simulink model "truck8_LQR00"  (Simulink 9.1)
settings: Solver=ode4  StartTime=0.0  StopTime=200  FixedStep=0.001  RelTol=1e-3  EnableMultiTasking=on
undefined symbols (not defined in the file): a1, a2, atable, atableall, cf_, cr_, den, dpsi, integrator_saturation_level1, integrator_saturation_level2, iz_, Kc, Kforward, Ki, ki1, ki2, KK1, KK2, KK3, KK4, KK_m2table, KK_vtable, Klon, kp1, kp2, Ksteer, lf_, londelay, lr_, m2, mass_, num, PP0, PP1, PP2, PP3, PP_m2table, PP_vtable, query_time, speed_controller_input_limit, st1, station_error_limit, steer0, steerdelay, t1, t2, Tlon, Tr, Tsteer, utable, utableall, v, vtable, wheelbase_
libraries: simulink x8, Solver_SF x1
settings Model: Creator=CIDI_xuhao  LastModifiedBy=DELL  SimulationMode=rapid-accelerator
settings DataIOCC: SaveFormat=Dataset
settings DebuggingCC: UnderspecifiedInitializationDetection=Simplified  MergeDetectMultiDrivingBlocksExec=error
settings HardwareCC: ProdBitPerPointer=64  ProdBitPerSizeT=64  ProdBitPerPtrDiffT=64  ProdLargestAtomicFloat=Float  ProdIntDivRoundTo=Zero  ProdEndianess=LittleEndian  ProdWordSize=64  ProdHWDeviceType=Intel->x86-64 (Windows64)
settings ModelReferenceCC: PropagateSignalLabelsOutOfModel=on
settings GRTTargetCC: GeneratePreprocessorConditionals=Disable all  CombineOutputUpdateFcns=on  GRTInterface=off

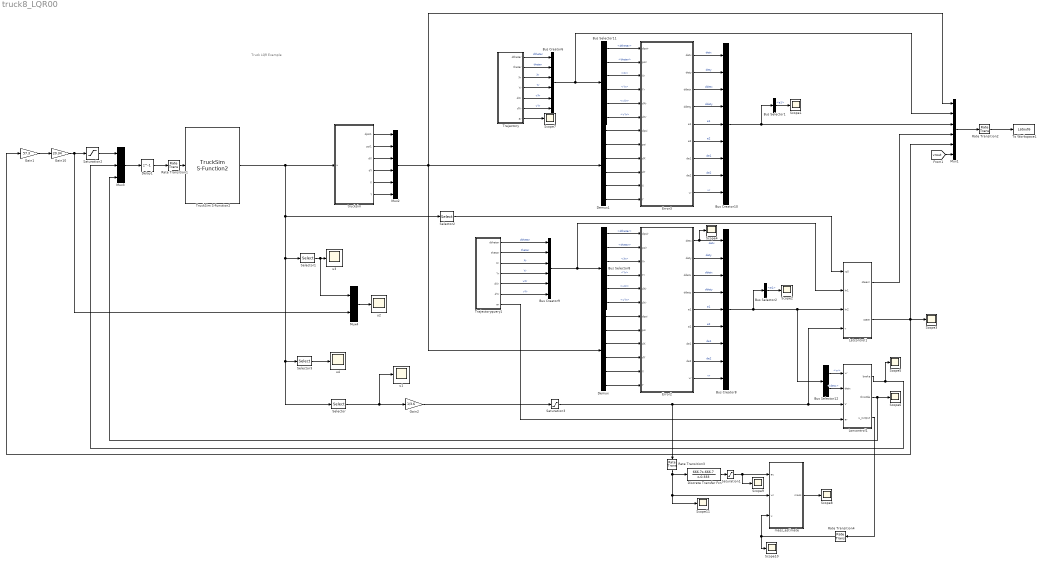
== system truck8_LQR00 ==
  note: Truck LQR Example
  Bus Creator10 : BusCreator  Inputs=9
  Bus Creator6 : BusCreator  Inputs=6
  Bus Creator8 : BusCreator  Inputs=9
  Bus Creator9 : BusCreator  Inputs=6
  Bus Selector1 : BusSelector  OutputSignals=e1
  Bus Selector11 : BusSelector  OutputSignals=dthetar,thetar,Xr,Yr,vXr,vYr
  Bus Selector12 : BusSelector  OutputSignals=vr,detx
  Bus Selector2 : BusSelector  OutputSignals=e1
  Bus Selector8 : BusSelector  OutputSignals=dthetar,thetar,Xr,Yr,vXr,vYr
  Delay1 : Delay  DelayLength=1  InitialCondition=0
  Demux : Demux  Outputs=6
  Demux1 : Demux  Outputs=6
  Discrete Transfer Fcn : DiscreteTransferFcn  Numerator=[666.7 -666.7]  Denominator=[1 -0.333]
  Error2 : MATLAB Function  TreatAsAtomicUnit=on
  Error3 : MATLAB Function  TreatAsAtomicUnit=on
  Gain1 : Gain  Gain=57.3
  Gain10 : Gain  Gain=20.34
  Gain2 : Gain  Gain=1/3.6
  Latcontrol1 : Subsystem
  Loncontrol1 : Subsystem
  Mux1 : Mux  Inputs=6
  Mux2 : Mux  Inputs=6
  Mux3 : Mux  Inputs=3
  Mux4 : Mux  Inputs=2
  Rate Transition1 : RateTransition  OutPortSampleTime=0.001
  Rate Transition2 : RateTransition  OutPortSampleTime=0.01
  Rate Transition3 : RateTransition  OutPortSampleTime=0.01
  Rate Transition4 : RateTransition  OutPortSampleTime=0.01
  Saturation1 : Saturate  UpperLimit=2  LowerLimit=-2
  Saturation2 : Saturate  UpperLimit=800  LowerLimit=-800
  Saturation3 : Saturate  UpperLimit=inf  LowerLimit=0.1
  Scope{1..11} (11 alike) : Scope
  Selector : Selector  InputPortWidth=13  IndexOptions=Index vector (dialog)  Indices=[4]  OutputSizes=1
  Selector1 : Selector  InputPortWidth=13  IndexOptions=Index vector (dialog)  Indices=[11 12]  OutputSizes=1
  Selector2 : Selector  InputPortWidth=13  IndexOptions=Index vector (dialog)  Indices=[11]  OutputSizes=1
  Selector3 : Selector  InputPortWidth=13  IndexOptions=Index vector (dialog)  Indices=[13]  OutputSizes=1
  To Workspace1 : ToWorkspace  VariableName=Latout6  SaveFormat=Timeseries  SampleTime=-1
  Trajectory : Subsystem
  Trajectoryquery1 : Subsystem
  TruckSim S-Function2 : Solver_SF/TruckSim S-Function2  Priority=1  VehicleCode=s_ss__sss  SIMFILE=simfile.sim
      settings: AttributesFormatString=Vehicle Code: %<VehicleCode>
  mass_estimate : Subsystem
  trucksim : MATLAB Function  TreatAsAtomicUnit=on
  u{1..4} (4 alike) : Scope
  wires:
  Selector/1 -> u1/1, Gain2/1
  Error2/7(de1) -> Bus Creator8/7  "de1"
  Trajectory/4(Yr) -> Bus Creator6/4  "Yr"
  Error2/3(ddetx) -> Bus Creator8/3  "ddetx"
  Bus Selector11/5 -> Error3/5(dXr)  "<vXr>"
  Demux/4 -> Error2/10(dY)
  Trajectoryquery1/1(dthetar) -> Bus Creator9/1  "dthetar"
  Error3/8(de2) -> Bus Creator10/8  "de2"
  Demux/1 -> Error2/7(dpsi)
  Error3/7(de1) -> Bus Creator10/7  "de1"
  Trajectoryquery1/5(dXr) -> Bus Creator9/5  "vXr"
  Bus Selector11/6 -> Error3/6(dYr)  "<vYr>"
  Bus Creator10/1 -> Bus Selector1/1, Mux1/3
  Error3/4(ddety) -> Bus Creator10/4  "ddety"
  Bus Selector12/1 -> Loncontrol1/1(vr)  "<vr>"
  Bus Selector11/3 -> Error3/3(Xr)  "<Xr>"
  Bus Selector11/2 -> Error3/2(psir)  "<thetar>"
  Demux1/6 -> Error3/12(Y)
  Bus Selector11/4 -> Error3/4(Yr)  "<Yr>"
  Error3/3(ddetx) -> Bus Creator10/3  "ddetx"
  Bus Selector12/2 -> Loncontrol1/2(detx)  "<detx>"
  Demux1/1 -> Error3/7(dpsi)
  [vrout] -> Mux1/6
  Bus Selector11/1 -> Error3/1(dpsir)  "<dthetar>"
  Demux1/5 -> Error3/11(X)
  Trajectoryquery1/6(dYr) -> Bus Creator9/6  "vYr"
  Error3/2(dety) -> Bus Creator10/2  "dety"
  Bus Selector8/2 -> Error2/2(psir)  "<thetar>"
  Error3/1(detx) -> Bus Creator10/1  "detx"
  Error2/5(e1) -> Bus Creator8/5  "e1"
  Demux/6 -> Error2/12(Y)
  Error3/6(e2) -> Bus Creator10/6  "e2"
  Error2/6(e2) -> Bus Creator8/6  "e2"
  Error3/9(vr) -> Bus Creator10/9  "vr"
  Demux/2 -> Error2/8(psi)
  Error2/2(dety) -> Bus Creator8/2  "dety"
  Error2/9(vr) -> Bus Creator8/9  "vr"
  Latcontrol1/1(steerc) -> Mux1/4
  Bus Selector8/3 -> Error2/3(Xr)  "<Xr>"
  Trajectoryquery1/2(thetar) -> Bus Creator9/2  "thetar"
  Bus Selector8/4 -> Error2/4(Yr)  "<Yr>"
  Bus Selector8/5 -> Error2/5(dXr)  "<vXr>"
  Error2/8(de2) -> Bus Creator8/8  "de2"
  Trajectory/5(dXr) -> Bus Creator6/5  "vXr"
  Trajectory/3(Xr) -> Bus Creator6/3  "Xr"
  Trajectory/6(dYr) -> Bus Creator6/6  "vYr"
  Trajectory/2(thetar) -> Bus Creator6/2  "thetar"
  Demux/3 -> Error2/9(dX)
  Bus Selector8/6 -> Error2/6(dYr)  "<vYr>"
  Error3/5(e1) -> Bus Creator10/5  "e1"
  Error2/1(detx) -> Bus Creator8/1, Scope4/1  "detx"
  Error2/4(ddety) -> Bus Creator8/4  "ddety"
  Mux1/1 -> Rate Transition2/1
  Bus Selector8/1 -> Error2/1(dpsir)  "<dthetar>"
  Trajectoryquery1/3(Xr) -> Bus Creator9/3  "Xr"
  Demux/5 -> Error2/11(X)
  Trajectoryquery1/4(Yr) -> Bus Creator9/4  "Yr"
  Trajectory/1(dthetar) -> Bus Creator6/1  "dthetar"
  Rate Transition2/1 -> To Workspace1/1
  Rate Transition1/1 -> TruckSim S-Function2/1
  trucksim/1(dpsi1) -> Mux2/1
  trucksim/2(psi1) -> Mux2/2
  trucksim/3(dX) -> Mux2/3
  trucksim/4(dY) -> Mux2/4
  trucksim/5(X) -> Mux2/5
  trucksim/6(Y) -> Mux2/6
  Demux1/2 -> Error3/8(psi)
  Demux1/3 -> Error3/9(dX)
  Demux1/4 -> Error3/10(dY)
  Bus Creator6/1 -> Bus Selector11/1, Mux1/2
  Mux2/1 -> Demux/1, Demux1/1, Mux1/1
  Selector1/1 -> Mux4/1, u3/1
  Bus Selector1/1 -> Scope1/1  "<e1>"
  Mux3/1 -> Delay1/1
  Loncontrol1/2(throttle) -> Scope6/1, Mux3/3
  Gain2/1 -> Saturation3/1
  Delay1/1 -> Rate Transition1/1
  Bus Selector2/1 -> Scope2/1  "<e1>"
  Loncontrol1/1(brake) -> Scope5/1, Mux3/2
  Trajectoryquery1/7(ar) -> Loncontrol1/4(ar)
  Trajectory/7(ar) -> Scope7/1
  TruckSim S-Function2/1 -> trucksim/1(u), Selector1/1, Selector3/1, Selector/1, Selector2/1
  Bus Creator9/1 -> Latcontrol1/2(In1), Bus Selector8/1
  Saturation3/1 -> Latcontrol1/4(v), Loncontrol1/3(V), Rate Transition3/1
  Bus Creator8/1 -> Latcontrol1/3(In2), Bus Selector12/1, Bus Selector2/1
  Latcontrol1/2(steer) -> Gain1/1, Scope3/1, Mux1/5
  Gain1/1 -> Gain10/1
  Gain10/1 -> Mux4/2, Saturation2/1
  Saturation2/1 -> Mux3/1
  Mux4/1 -> u2/1
  Selector2/1 -> Latcontrol1/1(roll)
  Selector3/1 -> u4/1
  mass_estimate/1(mass) -> Scope8/1
  Rate Transition3/1 -> Discrete Transfer Fcn/1, Scope11/1, mass_estimate/2(vc)
  Discrete Transfer Fcn/1 -> Saturation1/1
  Loncontrol1/3(u_output) -> Rate Transition4/1
  Rate Transition4/1 -> mass_estimate/3(u), Scope10/1
  Saturation1/1 -> Scope9/1, mass_estimate/1(ac)

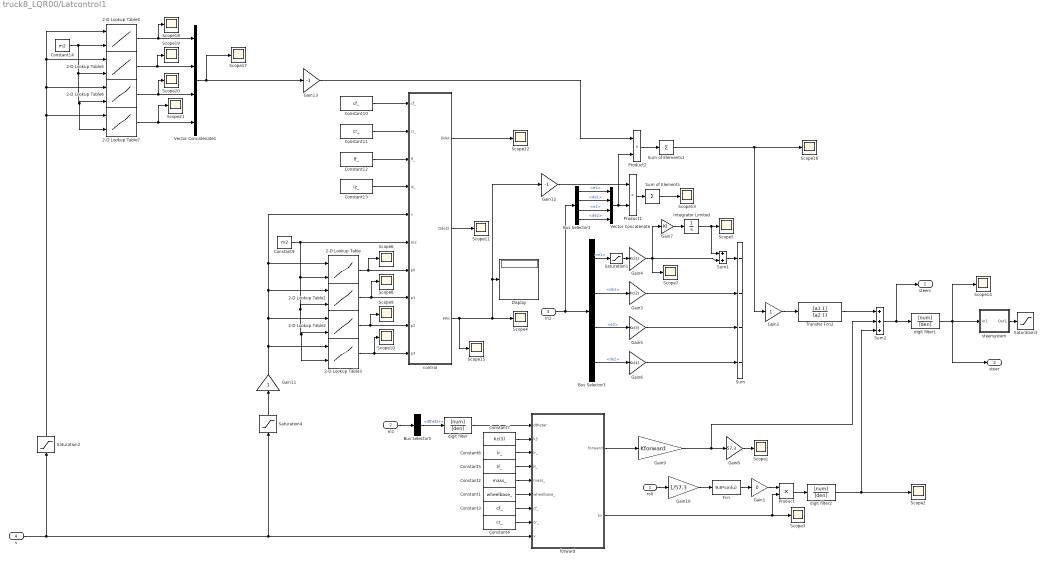
== system truck8_LQR00/Latcontrol1 ==
  roll : Inport
  In1 : Inport  Port=2
  In2 : Inport  Port=3
  v : Inport  Port=4
  2-D Lookup Table : Lookup_n-D  BreakpointsForDimension1=PP_vtable  BreakpointsForDimension2=PP_m2table  Table=PP0  ExtrapMethod=Clip  InternalRulePriority=Speed  RndMeth=Simplest  InputSameDT=on
  2-D Lookup Table1 : Lookup_n-D  BreakpointsForDimension1=PP_vtable  BreakpointsForDimension2=PP_m2table  Table=PP1  ExtrapMethod=Clip  InternalRulePriority=Speed  RndMeth=Simplest  InputSameDT=on
  2-D Lookup Table2 : Lookup_n-D  BreakpointsForDimension1=PP_vtable  BreakpointsForDimension2=PP_m2table  Table=PP2  ExtrapMethod=Clip  InternalRulePriority=Speed  RndMeth=Simplest  InputSameDT=on
  2-D Lookup Table3 : Lookup_n-D  BreakpointsForDimension1=PP_vtable  BreakpointsForDimension2=PP_m2table  Table=PP3  ExtrapMethod=Clip  InternalRulePriority=Speed  RndMeth=Simplest  InputSameDT=on
  2-D Lookup Table4 : Lookup_n-D  BreakpointsForDimension1=KK_vtable  BreakpointsForDimension2=KK_m2table  Table=KK1  ExtrapMethod=Clip  InternalRulePriority=Speed  RndMeth=Simplest  InputSameDT=on
  2-D Lookup Table5 : Lookup_n-D  BreakpointsForDimension1=KK_vtable  BreakpointsForDimension2=KK_m2table  Table=KK2  ExtrapMethod=Clip  InternalRulePriority=Speed  RndMeth=Simplest  InputSameDT=on
  2-D Lookup Table6 : Lookup_n-D  BreakpointsForDimension1=KK_vtable  BreakpointsForDimension2=KK_m2table  Table=KK3*1  ExtrapMethod=Clip  InternalRulePriority=Speed  RndMeth=Simplest  InputSameDT=on
  2-D Lookup Table7 : Lookup_n-D  BreakpointsForDimension1=KK_vtable  BreakpointsForDimension2=KK_m2table  Table=KK4  ExtrapMethod=Clip  InternalRulePriority=Speed  RndMeth=Simplest  InputSameDT=on
  Bus Selector1 : BusSelector  OutputSignals=e1,de1,e2,de2
  Bus Selector3 : BusSelector  OutputSignals=e1,de1,e2,de2
  Bus Selector5 : BusSelector  OutputSignals=dthetar
  Constant1 : Constant  Value=wheelbase_
  Constant10 : Constant  Value=cf_
  Constant11 : Constant  Value=cr_
  Constant12 : Constant  Value=lf_
  Constant13 : Constant  Value=iz_
  Constant14 : Constant  Value=m2
  Constant2 : Constant  Value=mass_
  Constant3 : Constant  Value=cf_
  Constant4 : Constant  Value=cr_
  Constant5 : Constant  Value=lf_
  Constant6 : Constant  Value=lr_
  Constant7 : Constant  Value=Kc(3)
  Constant9 : Constant  Value=m2
  Display : Display
  Fcn : Fcn  Expr=9.8*sin(u)
  Gain1 : Gain  Gain=0
  Gain10 : Gain  Gain=1/57.3
  Gain11 : Gain
  Gain12 : Gain  Gain=-1
  Gain13 : Gain  Gain=-1
  Gain2 : Gain
  Gain3 : Gain  Gain=Kc(2)
  Gain4 : Gain  Gain=Kc(1)
  Gain5 : Gain  Gain=Kc(3)
  Gain6 : Gain  Gain=Kc(4)
  Gain7 : Gain  Gain=Ki
  Gain8 : Gain  Gain=57.3
  Gain9 : Gain  Gain=Kforward
  Integrator Limited : Integrator  LimitOutput=on  UpperSaturationLimit=1  LowerSaturationLimit=-1
  Product : Product
  Product1 : Product
  Product2 : Product
  Saturation1 : Saturate  UpperLimit=10  LowerLimit=-10
  Saturation2 : Saturate  UpperLimit=25  LowerLimit=5/3.6
  Saturation3 : Saturate  UpperLimit=30/57.3  LowerLimit=-30/57.3
  Saturation4 : Saturate  UpperLimit=25  LowerLimit=10/3.6
  Scope{1..21} (21 alike) : Scope
  Sum : Sum  Inputs=----
  Sum of Elements : Sum  Inputs=+
  Sum of Elements1 : Sum  Inputs=+
  Sum1 : Sum
  Sum2 : Sum  Inputs=+++
  Transfer Fcn2 : TransferFcn  Numerator=[a1 1]  Denominator=[a2 1]
  Vector Concatenate : Concatenate  NumInputs=4
  Vector Concatenate1 : Concatenate  NumInputs=4
  control : MATLAB Function  TreatAsAtomicUnit=on
  digit filter : TransferFcn  Numerator=[num]  Denominator=[den]
  digit filter1 : TransferFcn  Numerator=[num]  Denominator=[den]
  digit filter2 : TransferFcn  Numerator=[num]  Denominator=[den]
  forward : MATLAB Function  TreatAsAtomicUnit=on
  steersystem : Subsystem
  steerc : Outport
  steer : Outport  Port=2
  wires:
  v/1 -> Saturation2/1, forward/9(v), Saturation4/1
  In2/1 -> Bus Selector1/1, Bus Selector3/1
  Bus Selector5/1 -> digit filter/1  "<dthetar>"
  In1/1 -> Bus Selector5/1
  Constant7/1 -> forward/2(k3)
  Gain8/1 -> Scope1/1
  forward/1(forward) -> Gain9/1
  Constant3/1 -> forward/7(cf_)
  Constant6/1 -> forward/3(lr_)
  Constant5/1 -> forward/4(lf_)
  Gain9/1 -> Sum2/2, Gain8/1
  Constant4/1 -> forward/8(cr_)
  steersystem/1(Out1) -> Saturation3/1
  Constant2/1 -> forward/5(mass_)
  Bus Selector3/2 -> Gain3/1  "<de1>"
  Bus Selector3/3 -> Gain5/1  "<e2>"
  Sum1/1 -> Sum/1
  Bus Selector3/1 -> Saturation1/1  "<e1>"
  Saturation1/1 -> Gain4/1
  Gain6/1 -> Sum/4
  Gain5/1 -> Sum/3
  Integrator Limited/1 -> Sum1/1, Scope5/1
  Gain4/1 -> Sum1/2, Scope7/1, Gain7/1
  Bus Selector3/4 -> Gain6/1  "<de2>"
  Constant1/1 -> forward/6(wheelbase_)
  Gain3/1 -> Sum/2
  Gain7/1 -> Integrator Limited/1
  digit filter/1 -> forward/1(dthetar)
  Gain2/1 -> Transfer Fcn2/1
  Sum2/1 -> steerc/1, digit filter1/1
  digit filter1/1 -> Scope14/1, steer/1, steersystem/1(In1)
  roll/1 -> Gain10/1
  Fcn/1 -> Gain1/1
  Gain10/1 -> Fcn/1
  digit filter2/1 -> Scope2/1, Sum2/3
  Gain1/1 -> Product/1
  Product/1 -> digit filter2/1
  forward/2(kv) -> Scope3/1, Product/2
  Transfer Fcn2/1 -> Sum2/1
  Constant12/1 -> control/3(lf_)
  Constant9/1 -> 2-D Lookup Table3/2, 2-D Lookup Table2/2, 2-D Lookup Table1/2, 2-D Lookup Table/2, control/6(m2)
  Constant10/1 -> control/1(cf_)
  Constant11/1 -> control/2(cr_)
  Constant13/1 -> control/4(iz_)
  2-D Lookup Table/1 -> Scope6/1, control/7(p0)
  2-D Lookup Table1/1 -> Scope8/1, control/8(p1)
  2-D Lookup Table3/1 -> Scope10/1, control/10(p3)
  Gain11/1 -> control/5(v), 2-D Lookup Table/1, 2-D Lookup Table1/1, 2-D Lookup Table2/1, 2-D Lookup Table3/1
  2-D Lookup Table2/1 -> Scope9/1, control/9(p2)
  Saturation4/1 -> Gain11/1
  control/2(Ddet2) -> Scope11/1
  control/1(Ddet) -> Scope12/1
  Bus Selector1/1 -> Vector Concatenate/1  "<e1>"
  Bus Selector1/2 -> Vector Concatenate/2  "<de1>"
  Bus Selector1/3 -> Vector Concatenate/3  "<e2>"
  Bus Selector1/4 -> Vector Concatenate/4  "<de2>"
  Vector Concatenate/1 -> Product2/2, Product1/2
  Product1/1 -> Sum of Elements/1
  Sum of Elements/1 -> Scope13/1
  Gain12/1 -> Product1/1
  control/3(PPK) -> Gain12/1, Display/1, Scope4/1, Scope15/1
  Saturation2/1 -> 2-D Lookup Table7/1, 2-D Lookup Table6/1, 2-D Lookup Table5/1, 2-D Lookup Table4/1
  2-D Lookup Table4/1 -> Scope18/1, Vector Concatenate1/1
  Constant14/1 -> 2-D Lookup Table4/2, 2-D Lookup Table5/2, 2-D Lookup Table7/2, 2-D Lookup Table6/2
  2-D Lookup Table5/1 -> Scope19/1, Vector Concatenate1/2
  2-D Lookup Table6/1 -> Scope20/1, Vector Concatenate1/3
  2-D Lookup Table7/1 -> Scope21/1, Vector Concatenate1/4
  Product2/1 -> Sum of Elements1/1
  Vector Concatenate1/1 -> Scope17/1, Gain13/1
  Sum of Elements1/1 -> Scope16/1, Gain2/1
  Gain13/1 -> Product2/1

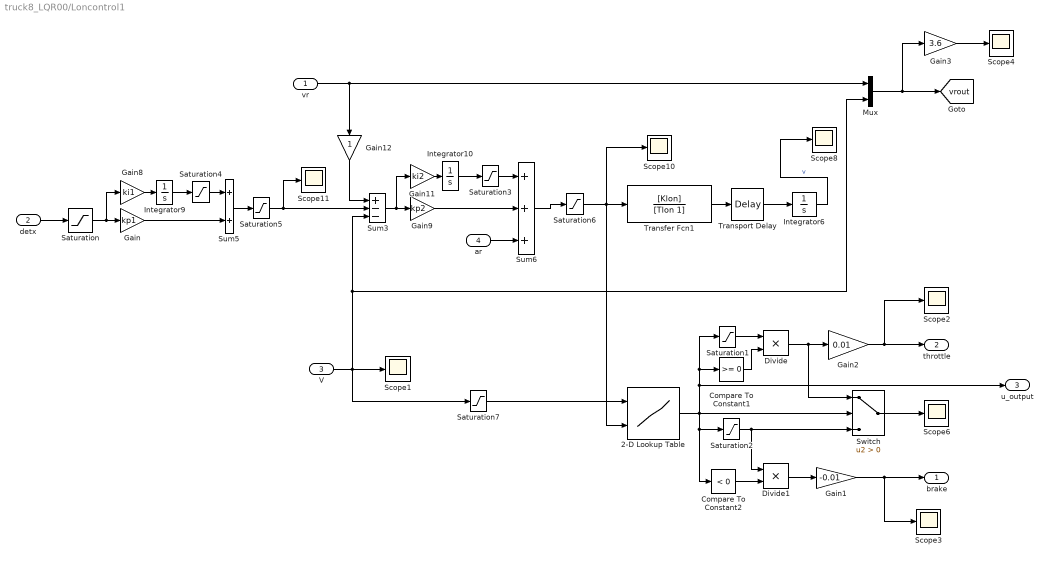
== system truck8_LQR00/Loncontrol1 ==
  vr : Inport
  detx : Inport  Port=2
  V : Inport  Port=3
  ar : Inport  Port=4
  2-D Lookup Table : Lookup_n-D  BreakpointsForDimension1=vtable  BreakpointsForDimension2=atable  Table=utableall  ExtrapMethod=Clip  InternalRulePriority=Speed  RndMeth=Simplest  InputSameDT=on
  Compare To Constant1 : simulink/Logic and Bit Operations/Compare To Constant  relop=>=  const=0  OutDataTypeStr=boolean
  Compare To Constant2 : simulink/Logic and Bit Operations/Compare To Constant  relop=<  const=0  OutDataTypeStr=boolean
  Divide : Product  Inputs=**
  Divide1 : Product  Inputs=**
  Gain : Gain  Gain=kp1
  Gain1 : Gain  Gain=-0.01
  Gain11 : Gain  Gain=ki2
  Gain12 : Gain
  Gain2 : Gain  Gain=0.01
  Gain3 : Gain  Gain=3.6
  Gain8 : Gain  Gain=ki1
  Gain9 : Gain  Gain=kp2
  Integrator10 : Integrator
  Integrator6 : Integrator
  Integrator9 : Integrator
  Mux : Mux  Inputs=2
  Saturation : Saturate  UpperLimit=station_error_limit  LowerLimit=-station_error_limit
  Saturation1 : Saturate  UpperLimit=90  LowerLimit=40*0.2
  Saturation2 : Saturate  UpperLimit=-30*0.2  LowerLimit=-60
  Saturation3 : Saturate  UpperLimit=integrator_saturation_level2  LowerLimit=-integrator_saturation_level2
  Saturation4 : Saturate  UpperLimit=integrator_saturation_level1  LowerLimit=-integrator_saturation_level1
  Saturation5 : Saturate  UpperLimit=speed_controller_input_limit  LowerLimit=-speed_controller_input_limit
  Saturation6 : Saturate  UpperLimit=5  LowerLimit=-5
  Saturation7 : Saturate  UpperLimit=100  LowerLimit=0.1
  Scope{1..4,6,8,10..11} (8 alike) : Scope
  Sum3 : Sum  Inputs=+--
  Sum5 : Sum
  Sum6 : Sum  Inputs=+++
  Switch : Switch  Criteria=u2 > Threshold
  Transfer Fcn1 : TransferFcn  Numerator=[Klon]  Denominator=[Tlon 1]
  Transport Delay : TransportDelay  DelayTime=londelay
  brake : Outport
  throttle : Outport  Port=2
  u_output : Outport  Port=3
  tag scope: vrout=global
  wires:
  Mux/1 -> Gain3/1, [vrout]
  detx/1 -> Saturation/1
  Integrator9/1 -> Saturation4/1
  Saturation3/1 -> Sum6/1
  Gain9/1 -> Sum6/2
  vr/1 -> Gain12/1, Mux/1
  Sum3/1 -> Gain11/1, Gain9/1
  Saturation/1 -> Gain/1, Gain8/1
  Gain8/1 -> Integrator9/1
  Saturation6/1 -> 2-D Lookup Table/2, Transfer Fcn1/1, Scope10/1
  Gain11/1 -> Integrator10/1
  Saturation5/1 -> Scope11/1, Sum3/2
  Gain/1 -> Sum5/2
  Integrator10/1 -> Saturation3/1
  Gain12/1 -> Sum3/1
  Saturation4/1 -> Sum5/1
  Transfer Fcn1/1 -> Transport Delay/1
  Sum5/1 -> Saturation5/1
  Transport Delay/1 -> Integrator6/1
  V/1 -> Sum3/3, Mux/2, Saturation7/1, Scope1/1
  Saturation2/1 -> Divide1/1, Switch/3
  Sum6/1 -> Saturation6/1
  Switch/1 -> Scope6/1
  Integrator6/1 -> Scope8/1  "v"
  Saturation7/1 -> 2-D Lookup Table/1
  Gain2/1 -> Scope2/1, throttle/1
  Gain1/1 -> Scope3/1, brake/1
  2-D Lookup Table/1 -> u_output/1, Compare To Constant1/1, Saturation1/1, Switch/2, Compare To Constant2/1, Saturation2/1
  Saturation1/1 -> Divide/1
  Compare To Constant1/1 -> Divide/2
  Divide/1 -> Gain2/1, Switch/1
  Compare To Constant2/1 -> Divide1/2
  Divide1/1 -> Gain1/1
  ar/1 -> Sum6/3
  Gain3/1 -> Scope4/1

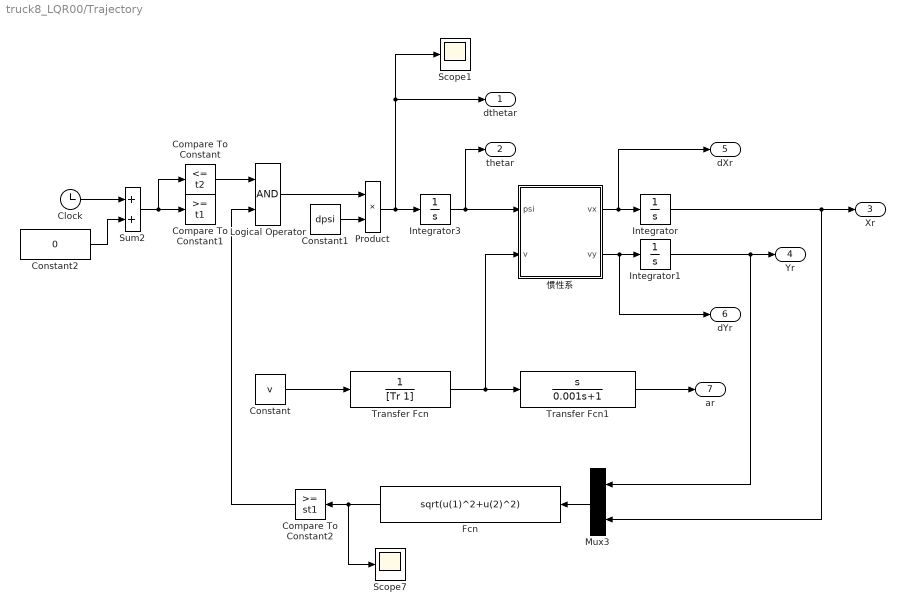
== system truck8_LQR00/Trajectory ==
  Clock : Clock
  Compare To Constant : simulink/Logic and Bit Operations/Compare To Constant  relop=<=  const=t2  OutDataTypeStr=boolean
  Compare To Constant1 : simulink/Logic and Bit Operations/Compare To Constant  relop=>=  const=t1  OutDataTypeStr=boolean
  Compare To Constant2 : simulink/Logic and Bit Operations/Compare To Constant  relop=>=  const=st1  OutDataTypeStr=boolean
  Constant : Constant  Value=v
  Constant1 : Constant  Value=dpsi
  Constant2 : Constant  Value=0
  Fcn : Fcn  Expr=sqrt(u(1)^2+u(2)^2)
  Integrator : Integrator
  Integrator1 : Integrator
  Integrator3 : Integrator
  Logical Operator : Logic  AllPortsSameDT=off  OutDataTypeStr=boolean
  Mux3 : Mux  Inputs=2
  Product : Product
  Scope1 : Scope
  Scope7 : Scope
  Sum2 : Sum
  Transfer Fcn : TransferFcn  Denominator=[Tr 1]
  Transfer Fcn1 : TransferFcn  Numerator="[1  0]"  Denominator=[0.001 1]
  惯性系 : MATLAB Function  TreatAsAtomicUnit=on
  dthetar : Outport
  thetar : Outport  Port=2
  Xr : Outport  Port=3
  Yr : Outport  Port=4
  dXr : Outport  Port=5
  dYr : Outport  Port=6
  ar : Outport  Port=7
  wires:
  Compare To Constant2/1 -> Logical Operator/2
  Fcn/1 -> Scope7/1, Compare To Constant2/1
  Mux3/1 -> Fcn/1
  Transfer Fcn1/1 -> ar/1
  Transfer Fcn/1 -> 惯性系/2(v), Transfer Fcn1/1
  Integrator1/1 -> Yr/1, Mux3/1
  Integrator/1 -> Xr/1, Mux3/2
  Logical Operator/1 -> Product/1
  惯性系/2(vy) -> Integrator1/1, dYr/1
  Integrator3/1 -> thetar/1, 惯性系/1(psi)
  Constant/1 -> Transfer Fcn/1
  惯性系/1(vx) -> dXr/1, Integrator/1
  Compare To Constant/1 -> Logical Operator/1
  Constant1/1 -> Product/2
  Clock/1 -> Sum2/1
  Sum2/1 -> Compare To Constant/1, Compare To Constant1/1
  Constant2/1 -> Sum2/2
  Product/1 -> Scope1/1, dthetar/1, Integrator3/1

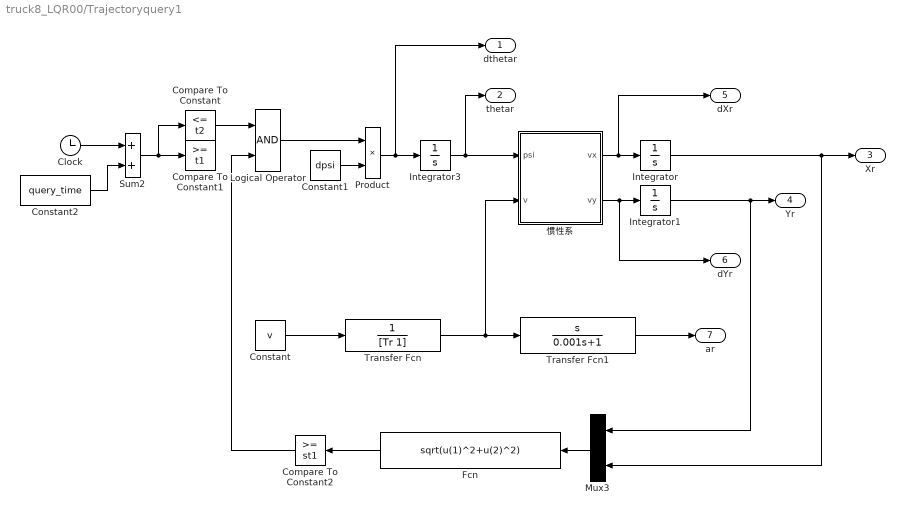
== system truck8_LQR00/Trajectoryquery1 ==
  Clock : Clock
  Compare To Constant : simulink/Logic and Bit Operations/Compare To Constant  relop=<=  const=t2  OutDataTypeStr=boolean
  Compare To Constant1 : simulink/Logic and Bit Operations/Compare To Constant  relop=>=  const=t1  OutDataTypeStr=boolean
  Compare To Constant2 : simulink/Logic and Bit Operations/Compare To Constant  relop=>=  const=st1  OutDataTypeStr=boolean
  Constant : Constant  Value=v
  Constant1 : Constant  Value=dpsi
  Constant2 : Constant  Value=query_time
  Fcn : Fcn  Expr=sqrt(u(1)^2+u(2)^2)
  Integrator : Integrator
  Integrator1 : Integrator
  Integrator3 : Integrator
  Logical Operator : Logic  AllPortsSameDT=off  OutDataTypeStr=boolean
  Mux3 : Mux  Inputs=2
  Product : Product
  Sum2 : Sum
  Transfer Fcn : TransferFcn  Denominator=[Tr 1]
  Transfer Fcn1 : TransferFcn  Numerator="[1  0]"  Denominator=[0.001 1]
  惯性系 : MATLAB Function  TreatAsAtomicUnit=on
  dthetar : Outport
  thetar : Outport  Port=2
  Xr : Outport  Port=3
  Yr : Outport  Port=4
  dXr : Outport  Port=5
  dYr : Outport  Port=6
  ar : Outport  Port=7
  wires:
  Constant2/1 -> Sum2/2
  Sum2/1 -> Compare To Constant1/1, Compare To Constant/1
  Clock/1 -> Sum2/1
  Constant1/1 -> Product/2
  Compare To Constant/1 -> Logical Operator/1
  惯性系/1(vx) -> Integrator/1, dXr/1
  Constant/1 -> Transfer Fcn/1
  Integrator3/1 -> 惯性系/1(psi), thetar/1
  惯性系/2(vy) -> dYr/1, Integrator1/1
  Logical Operator/1 -> Product/1
  Integrator/1 -> Mux3/2, Xr/1
  Product/1 -> Integrator3/1, dthetar/1
  Integrator1/1 -> Mux3/1, Yr/1
  Transfer Fcn/1 -> Transfer Fcn1/1, 惯性系/2(v)
  Transfer Fcn1/1 -> ar/1
  Mux3/1 -> Fcn/1
  Fcn/1 -> Compare To Constant2/1
  Compare To Constant2/1 -> Logical Operator/2

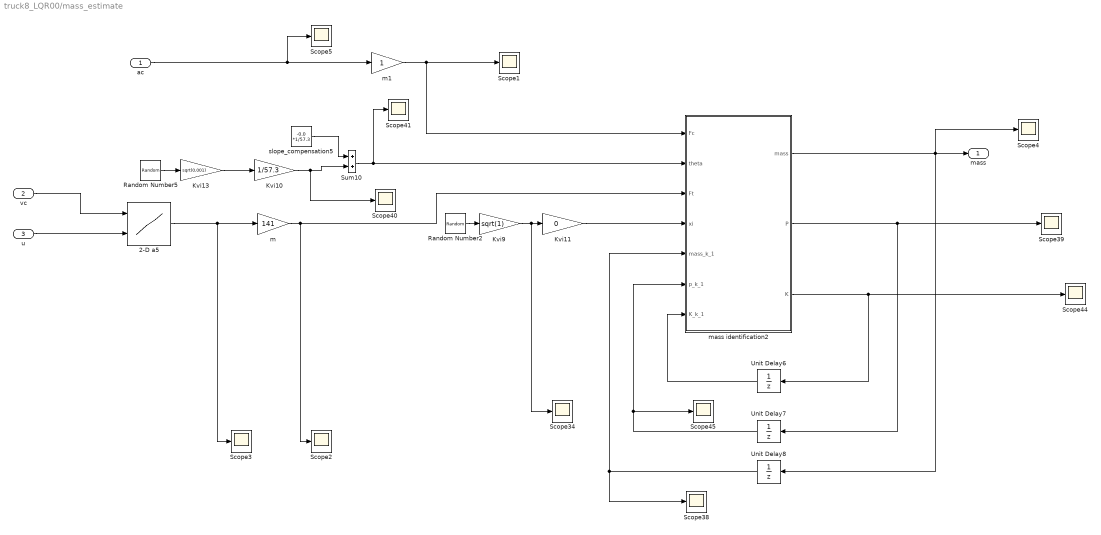
== system truck8_LQR00/mass_estimate ==
  ac : Inport
  vc : Inport  Port=2
  u : Inport  Port=3
  2-D a5 : Lookup_n-D  BreakpointsForDimension1=vtable  BreakpointsForDimension2=utable  BreakpointsForDimension3=[-60 -50]  Table=atableall  InternalRulePriority=Speed  RndMeth=Simplest  InputSameDT=on
  Kvi10 : Gain  Gain=1/57.3
  Kvi11 : Gain  Gain=0
  Kvi13 : Gain  Gain=sqrt(0.001)
  Kvi9 : Gain  Gain=sqrt(1)
  Random Number2 : RandomNumber  SampleTime=0.01
  Random Number5 : RandomNumber  Variance=0.1  SampleTime=0.01
  Scope{1..5,34,38..41,44..45} (12 alike) : Scope
  Sum10 : Sum
  Unit Delay6 : UnitDelay  InitialCondition=1  SampleTime=0.01
  Unit Delay7 : UnitDelay  InitialCondition=100000  SampleTime=0.01
  Unit Delay8 : UnitDelay  InitialCondition=30000  SampleTime=0.01
  m : Gain  Gain=141
  m1 : Gain
  mass identification2 : MATLAB Function  TreatAsAtomicUnit=on  SystemSampleTime=0.01
  slope_compensation5 : Constant  Value=-0.0 *1/57.3
  mass : Outport
  wires:
  Unit Delay7/1 -> mass identification2/6(p_k_1), Scope45/1
  mass identification2/1(mass) -> Scope4/1, Unit Delay8/1, mass/1
  mass identification2/3(K) -> Unit Delay6/1, Scope44/1
  Unit Delay6/1 -> mass identification2/7(K_k_1)
  Kvi13/1 -> Kvi10/1
  ac/1 -> Scope5/1, m1/1
  Kvi11/1 -> mass identification2/4(xi)
  Random Number2/1 -> Kvi9/1
  Unit Delay8/1 -> mass identification2/5(mass_k_1), Scope38/1
  slope_compensation5/1 -> Sum10/1
  Kvi10/1 -> Sum10/2, Scope40/1
  Random Number5/1 -> Kvi13/1
  mass identification2/2(P) -> Unit Delay7/1, Scope39/1
  2-D a5/1 -> Scope3/1, m/1
  vc/1 -> 2-D a5/1
  Kvi9/1 -> Kvi11/1, Scope34/1
  Sum10/1 -> mass identification2/2(theta), Scope41/1
  m/1 -> Scope2/1, mass identification2/3(Ft)
  u/1 -> 2-D a5/2
  m1/1 -> Scope1/1, mass identification2/1(Fc)

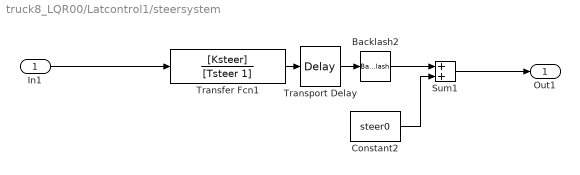
== system truck8_LQR00/Latcontrol1/steersystem ==
  In1 : Inport
  Backlash2 : Backlash  BacklashWidth=backlash
  Constant2 : Constant  Value=steer0
  Sum1 : Sum
  Transfer Fcn1 : TransferFcn  Numerator=[Ksteer]  Denominator=[Tsteer 1]
  Transport Delay : TransportDelay  DelayTime=steerdelay
  Out1 : Outport
  wires:
  Sum1/1 -> Out1/1
  Backlash2/1 -> Sum1/1
  In1/1 -> Transfer Fcn1/1
  Constant2/1 -> Sum1/2
  Transfer Fcn1/1 -> Transport Delay/1
  Transport Delay/1 -> Backlash2/1

== matlab function trucksim ==
  data: dpsi1 output double; u input double; psi1 output double; dX output double; dY output double; X output double; Y output double
function [dpsi1,psi1,dX,dY,X,Y]  = fcn(u)

%牵引车信息
X=u(1);
Y=u(2);
Yaw=u(3);
vx=u(4)/3.6;
vy=u(5)/3.6;
Avz=u(6);
      
%半挂车信息
X2=u(7);
Y2=u(8);
Yaw2=u(9);
Avz2=u(10);

roll=u(11);
roll2=u(12);
hitch=u(13);

% 车辆坐标系到大地坐标系的转换
psi1=Yaw/57.3;
dpsi1=Avz/57.3;

L=[cos(psi1) -sin(psi1);
      sin(psi1) cos(psi1)];

dX=vx*cos(psi1)-vy*sin(psi1);
dY=vx*sin(psi1)+vy*cos(psi1);%大地系下的速度

== matlab function Trajectory/惯性系 ==
  data: psi input double; vx output double; v input double; vy output double
function [vx,vy] = fcn(psi,v)

vx = v*cos(psi);
vy = v*sin(psi);

== matlab function Latcontrol1/control ==
  data: Ddet output double; Ddet2 output double; PPK output double; cf_ input double; cr_ input double; lf_ input double; iz_ input double; v input double; m2 input double; p0 input double; p1 input double; p2 input double; p3 input double
function [Ddet,Ddet2,PPK]= fcn(cf_,cr_,lf_,iz_,v,m2,p0,p1,p2,p3)

        C1 = cf_;
        C2 = cr_;
        C3 = cr_;
        C4 = cr_;
        C5 = cr_;
        C6 = cr_;
%         # Distance of each axle to COG
        l1 = lf_;
        l2 = lf_;
        l3 = l2+1.310;
        l4 = 4.400*0.85;
        l5 = l4+1.310;
        l6 = l5+1.310;
%         # Mass of each body
        m1 = 10000;
        mass_fl= 3000;
        mass_fr= 3000;
        mass_rl= 2000;
        mass_rr= 2000;
%         # Distance of hitch to COG for each body
        hF = (l2+l3)/2;
        hR = 7.16-4.4*0.85; %# approximation of hitch-COG distance of trailer
%         # Inertia moment of each body
        m1_f = mass_fl + mass_fr;
        m1_r = mass_rl + mass_rr;
        m2_f = m2*0.25;
        m2_r = m2*0.75; %# assume the rear wheelbases carry 75% of the weight
%         i1 = m1_f*l1*l1 + m1_r*hF*hF;
        i1 =iz_;
        i2 = m2_f*hR*hR + m2_r*l5*l5;
        
        matrix_a6_=zeros(6, 6);      
        matrix_b6_=zeros(6, 1);
        matrix_b6_2_=zeros(6, 1);   
        
        %
                
        Mm11=1;
        Mm22=m1+m2;
        Mm24=-m2*hF;
        Mm26=-m2*hR;
        Mm33=1;
        Mm42=-hF*m2;
        Mm44=i1+hF^2*m2;
        Mm46=hR*hF*m2;
        Mm55=1;
        Mm62=-hR*m2;
        Mm64=hF*hR*m2;
        Mm66=i2+hR^2*m2;
                
        aa11=-(C1+C2+C3)/v;
        aa12=(-C1*l1+C2*l2+C3*l3)/v-m1*v;
        aa13=-(C4+C5+C6)/v;
        aa14=(C4*l4+C5*l5+C6*l6)/v-m2*v;
        aa21=(-C1*l1+C2*l2+C3*l3)/v;
        aa22=(-C1*l1^2-C2*l2^2-C3*l3^2)/v;
        aa23=hF*(C4+C5+C6)/v;
        aa24=-hF*(C4*l4+C5*l5+C6*l6)/v+hF*m2*v;
        aa31=0;
        aa32=0;
        aa33=(hR*(C4+C5+C6)+C4*l4+C5*l5+C6*l6)/v;
        aa34=-(C4*l4*(l4+hR)+C5*l5*(l5+hR)+C6*l6*(l6+hR))/v+hR*m2*v;
        
        Mg3=zeros(6, 6);   
        Ag3=zeros(6, 6);   
        
        Mg3(1,1)=Mm11;
        Mg3(2,2)=Mm22;
        Mg3(2,4)=Mm24;
        Mg3(2,6)=Mm26;
        Mg3(3,3)=Mm33;
        Mg3(4,2)=Mm42;
        Mg3(4,4)=Mm44;
        Mg3(4,6)=Mm46;
        Mg3(5,5)=Mm55;
        Mg3(6,2)=Mm62;
        Mg3(6,4)=Mm64;
        Mg3(6,6)=Mm66;
        

        Ag3(1,2)=1;
        Ag3(2,2)=aa11+aa13;
        Ag3(2,3)=aa13*v;
        Ag3(2,4)=aa12-aa13*hF-m2*v;
        Ag3(2,5)=-aa13*v;
        Ag3(2,6)=aa14-aa13*hR+m2*v;
        Ag3(3,4)=1;
        Ag3(4,2)=aa21+aa23;
        Ag3(4,3)=aa23*v;
        Ag3(4,4)=aa22-aa23*hF+hF*m2*v;
        Ag3(4,5)=-aa23*v;
        Ag3(4,6)=aa24-aa23*hR-hF*m2*v;    
        Ag3(5,6)=1;   
        Ag3(6,2)=aa33;   
        Ag3(6,3)=aa33*v; 
        Ag3(6,4)=-aa33*hF+hR*m2*v; 
        Ag3(6,5)=-aa33*v; 
        Ag3(6,6)=aa34-aa33*hR-hR*m2*v; 

        Bg3=[0;C1;0;C1*l1;0;0];
        
        PPPem=eye(6);
        PPPem(6,4)=1;
        PPPem(6,6)=-1;
  
        PPPea=eye(6);
        PPPea(5,3)=1;
        PPPea(5,5)=-1;
        PPPea(6,4)=1;
        PPPea(6,6)=-1;
        
        
        Mgg3=Mg3*PPPem;
        Agg3=Ag3;
        Agg3(:,[1 2])=Ag3(:,[1 2]);
        Agg3(:,[3 4])=Ag3(:,[3  4])+Ag3(:,[5 6]);
        Agg3(5,4)=0;
        Agg3(:,[5 6])=-Ag3(:,[5 6]);
        Agg3(5,6)=1;
        
        Ag=Mgg3\Agg3;
        Bg=Mgg3\Bg3;
        
        
        matrix_a_6=Ag;
        matrix_a_6(2,3)=-Ag(2,2)*v;
        matrix_a_6(4,3)=-Ag(4,2)*v;
        matrix_a_6(6,3)=-Ag(6,2)*v;
        matrix_a_6(2,4)=Ag(2,4)+v;

        matrix_b_6=Bg;
        matrix_b_62=[0;Ag(2,4);0;Ag(4,4);0;Ag(6,4)];
        
        
a22=matrix_a_6(2,2);
a23=matrix_a_6(2,3);
a24=matrix_a_6(2,4);
a42=matrix_a_6(4,2);
a43=matrix_a_6(4,3);
a44=matrix_a_6(4,4);

b2=matrix_b_6(2);
b4=matrix_b_6(4);

     %s^4 
%      + (b2*k2 - a44 - a22 + b4*k4)*s^3 
%      + (a22*a44 - a43 - a24*a42 + b2*k1 + b4*k3 - a22*b4*k4 + a24*b4*k2 + a42*b2*k4 - a44*b2*k2)*s^2
%      + (a22*a43 - a23*a42 - a22*b4*k3 + a23*b4*k2 + a24*b4*k1 + a42*b2*k3 - a43*b2*k2 - a44*b2*k1)*s 
%      + a23*b4*k1 - a43*b2*k1

d1=(a23*b4- a43*b2);
d2=a24*b4- a44*b2;
d3=a42*b2- a22*b4;
d4=b2;
d5=b4;


D =[ d1,  0,  0,  0
        d2, d1, d3,  0
        d4, d2, d5, d3
        0, d4,  0, d5];
    
Ddet=   (d1*(d4*d3^2 - d2*d3*d5 + d1*d5^2));
Ddet2=(d4*d3^2 - d2*d3*d5 + d1*d5^2);

if abs(Ddet)<100
    Ddet=100*sign(Ddet);
end

if abs(Ddet2)<1
    Ddet2=100*sign(Ddet2);
end

    
invD=[                      1/d1,                                                        0,                                     0,                                       0;
              -(d5*(d2*d5 - d3*d4))/Ddet,                             d5^2/Ddet2,                   -(d3*d5)/Ddet2,                d3^2/Ddet2;
        -(- d5*d2^2 + d3*d4*d2 + d1*d4*d5)/Ddet,        -(d2*d5 - d3*d4)/Ddet2,     (d1*d5)/Ddet2,              -(d1*d3)/Ddet2;
              -(d3*d4^2 - d2*d5*d4)/Ddet,                        -(d4*d5)/Ddet2,                  (d3*d4)/Ddet2,          -(d2*d3 - d1*d5)/Ddet2];  
PPK=invD*[p0;p1-(a22*a43 - a23*a42 );p2-(a22*a44 - a43 - a24*a42 );p3-( - a44 - a22 )];%得到k1,k2,k3,k4
% PPK=D\[p0;p1-(a22*a43 - a23*a42 );p2-(a22*a44 - a43 - a24*a42 );p3-( - a44 - a22 )];%得到k1,k2,k3,k4

== matlab function mass_estimate/mass identification2 ==
  data: mass output double; Fc input double; theta input double; Ft input double; xi input double; mass_k_1 input double; p_k_1 input double; K_k_1 input double; P output double; K output double
function [mass,P,K] = fcn(Fc,theta,Ft,xi,mass_k_1,p_k_1,K_k_1)
% Fc = 0;theta = 0;Ft = 0;
na = 1;nb = 1;d = 3; %structure parameters
uk = 0;%initial value of system input
yk = 0;%initial value of system output
L = 1;
g = 9.8;%unit:m/s^2
w = 0.998;
%theta = 0;% slope of the road,unit:degree or rad?

% xi = sqrt(0.1) * randn(L,1);%white noise 
if theta >= 0 
    i = -sin(theta); 
else
    i = sin(theta); 
end
% i = -sin(theta); 
phi = g * i;

Fg = (Fc - Ft - xi) * -1;
% mass = 0;% initial value of the object to be estimated
% persistent mass_last;
% mass_last = 0;
% P = 10^6 * eye(na - 1 + nb - 1 + 1);
% Fg = phi * m + xi; % y(k) = phi(k)' * theta + xi 标准的最小二乘形式
% mass_data 

% RLS algorithm
K = p_k_1 * phi / (w + phi' * p_k_1 * phi);
% mass = mass_last + K * (Fg - phi' * mass_last);
mass = mass_k_1 + K * (Fg - phi' * mass_k_1);
P =1 / w * (eye(na - 1 + nb - 1 + 1) - K * phi') * p_k_1;

% mass_last = mass;

== matlab function Error2 ==
  data: detx output double; dety output double; ddetx output double; ddety output double; e1 output double; e2 output double; dpsir input double; psir input double; Xr input double; Yr input double; dXr input double; dYr input double; dpsi input double; psi input double; dX input double; dY input double; X input double; Y input double; de1 output double; de2 output double; vr output double
function [detx,dety,ddetx,ddety,e1,e2,de1,de2,vr]   = fcn(dpsir,psir,Xr,Yr,dXr,dYr,dpsi,psi,dX,dY,X,Y)

vr=sqrt(dXr^2+dYr^2);
de2=dpsi-dpsir;

detX=X-Xr;
detY=Y-Yr;%惯性系下的偏差

ddetX=dX-dXr;
ddetY=dY-dYr;%车辆系下的偏差速度

ddetx=ddetX*cos(psi)+ddetY*sin(psi);
ddety=-ddetX*sin(psi)+ddetY*cos(psi);%车辆系下的偏差速度

vx=sqrt(dX^2+dY^2);
de1=vx*sin(psi-psir);

% detx=detX*cos(psi)+detY*sin(psi);
% dety=-detX*sin(psi)+detY*cos(psi);%惯性系转速度系下的偏差

detx=detX*cos(psir)+detY*sin(psir);
dety=-detX*sin(psir)+detY*cos(psir);%惯性系转速度系下的偏差

e1=dety;
e2=psi-psir;

== matlab function Error3 ==
  data: detx output double; dety output double; ddetx output double; ddety output double; e1 output double; e2 output double; dpsir input double; psir input double; Xr input double; Yr input double; dXr input double; dYr input double; dpsi input double; psi input double; dX input double; dY input double; X input double; Y input double; de1 output double; de2 output double; vr output double
function [detx,dety,ddetx,ddety,e1,e2,de1,de2,vr]   = fcn(dpsir,psir,Xr,Yr,dXr,dYr,dpsi,psi,dX,dY,X,Y)

vr=sqrt(dXr^2+dYr^2);
de2=dpsi-dpsir;

detX=X-Xr;
detY=Y-Yr;%惯性系下的偏差

ddetX=dX-dXr;
ddetY=dY-dYr;%车辆系下的偏差速度

ddetx=ddetX*cos(psi)+ddetY*sin(psi);
ddety=-ddetX*sin(psi)+ddetY*cos(psi);%车辆系下的偏差速度

vx=sqrt(dX^2+dY^2);
de1=vx*sin(psi-psir);

% detx=detX*cos(psi)+detY*sin(psi);
% dety=-detX*sin(psi)+detY*cos(psi);%惯性系转速度系下的偏差

detx=detX*cos(psir)+detY*sin(psir);
dety=-detX*sin(psir)+detY*cos(psir);%惯性系转速度系下的偏差

e1=dety;
e2=psi-psir;

== matlab function Latcontrol1/forward ==
  data: forward output double; dthetar input double; k3 input double; lr_ input double; lf_ input double; mass_ input double; wheelbase_ input double; cf_ input double; cr_ input double; v input double; kv output double
function [forward,kv]= fcn(dthetar,k3,lr_,lf_,mass_,wheelbase_,cf_,cr_,v)

ref_curvature=wheelbase_*dthetar/v;
kv =lr_ * mass_ / 2 / cf_ / wheelbase_ - lf_ * mass_ / 2 / cr_ / wheelbase_;

forward =(wheelbase_ * ref_curvature + kv * v * v * ref_curvature -k3*(lr_ * ref_curvature -lf_ * mass_ * v * v * ref_curvature / 2 / cr_ / wheelbase_)) ;

== matlab function Trajectoryquery1/惯性系 ==
  data: psi input double; vx output double; v input double; vy output double
function [vx,vy] = fcn(psi,v)

vx = v*cos(psi);
vy = v*sin(psi);
